simulink model "blockdemo"  (Simulink 6.3)
settings: Solver=VariableStepDiscrete  StartTime=0  StopTime=100  FixedStep=1  MaxStep=1  RelTol=1e-3
InitFcn:
  | %% DSPBuilder Start
  | alt_dspbuilder_update_model(bdroot)
  | %% DSPBuilder End
libraries: allblocks_alteradspbuilder2 x9, simulink x1
settings Model: Creator=mjervis  LastModifiedBy=delphick
settings DebuggingCC: MultiTaskDSMMsg=error

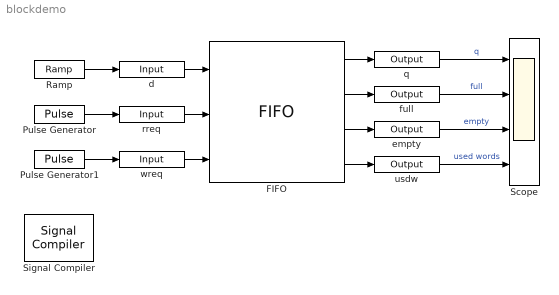
== system blockdemo ==
  FIFO : allblocks_alteradspbuilder2/FIFO  numwords=8  BusType=Inferred  bwl=8  bwr=0  ram_type=AUTO  use_sclr=off  use_les_only=off  showahead_mode=on
      settings: AttributesFormatString=Show-ahead Mode = %<showahead_mode>\nNumber of words = %<numwords>
  Pulse Generator : DiscretePulseGenerator  Period=30  PulseWidth=10  PhaseDelay=10
  Pulse Generator1 : DiscretePulseGenerator  Period=30  PulseWidth=10
  Ramp : simulink/Sources/Ramp  slope=1  start=0  X0=0
  Scope : Scope  NumInputPorts=4
      settings: TimeRange=100  YMin=-5~-0.5~-0.5~-2  YMax=20~1.5~1.5~8
  Signal Compiler : allblocks_alteradspbuilder2/Signal Compiler  DeviceFamily=Stratix III  DeviceName=AUTO  EnableSignalTap=off  SignalTapDepth=128  UseBoardBlock=off  StpUseDefaultClock=on  StpClock=clock
  d : allblocks_alteradspbuilder2/Input  iofile=C:\workspace_clean\Documentation\DesignExamples\Tutorials\UnitBlocks\Storage\FIFO\tb_blockdemo\blockdemo_d.salt  BusType=Unsigned Integer  bwl=4  bwr=0  SpecifyClock=off  PORTTYPE=Input
      settings: AttributesFormatString=%<BusType>
  empty : allblocks_alteradspbuilder2/Output  iofile=C:\workspace_clean\Documentation\DesignExamples\Tutorials\UnitBlocks\Storage\FIFO\tb_blockdemo\blockdemo_empty.capture  BusType=Single Bit  bwl=8  bwr=0  PORTTYPE=Output
  full : allblocks_alteradspbuilder2/Output  iofile=C:\workspace_clean\Documentation\DesignExamples\Tutorials\UnitBlocks\Storage\FIFO\tb_blockdemo\blockdemo_full.capture  BusType=Single Bit  bwl=8  bwr=0  PORTTYPE=Output
  q : allblocks_alteradspbuilder2/Output  iofile=C:\workspace_clean\Documentation\DesignExamples\Tutorials\UnitBlocks\Storage\FIFO\tb_blockdemo\blockdemo_q.capture  BusType=Inferred  bwl=8  bwr=0  PORTTYPE=Output
  rreq : allblocks_alteradspbuilder2/Input  iofile=C:\workspace_clean\Documentation\DesignExamples\Tutorials\UnitBlocks\Storage\FIFO\tb_blockdemo\blockdemo_rreq.salt  BusType=Single Bit  bwl=4  bwr=0  SpecifyClock=off  PORTTYPE=Input
  usdw : allblocks_alteradspbuilder2/Output  iofile=C:\workspace_clean\Documentation\DesignExamples\Tutorials\UnitBlocks\Storage\FIFO\tb_blockdemo\blockdemo_usdw.capture  BusType=Unsigned Integer  bwl=3  bwr=0  PORTTYPE=Output
  wreq : allblocks_alteradspbuilder2/Input  iofile=C:\workspace_clean\Documentation\DesignExamples\Tutorials\UnitBlocks\Storage\FIFO\tb_blockdemo\blockdemo_wreq.salt  BusType=Single Bit  bwl=4  bwr=0  SpecifyClock=off  PORTTYPE=Input
  wires:
  d/1 -> FIFO/1
  FIFO/1 -> q/1
  rreq/1 -> FIFO/2
  wreq/1 -> FIFO/3
  FIFO/2 -> full/1
  FIFO/4 -> usdw/1
  FIFO/3 -> empty/1
  Ramp/1 -> d/1
  Pulse Generator/1 -> rreq/1
  Pulse Generator1/1 -> wreq/1
  q/1 -> Scope/1  "q"
  full/1 -> Scope/2  "full"
  empty/1 -> Scope/3  "empty"
  usdw/1 -> Scope/4  "used words"
